simulink model "modellosimulink_sparo"  (R2024b)
settings: Solver=VariableStepAuto  StartTime=0.0  StopTime=10.0  RelTol=1e-3
libraries: arduinolib x29
settings Model: Creator=Andrea Blumer  LastModifiedBy=Andrea Blumer

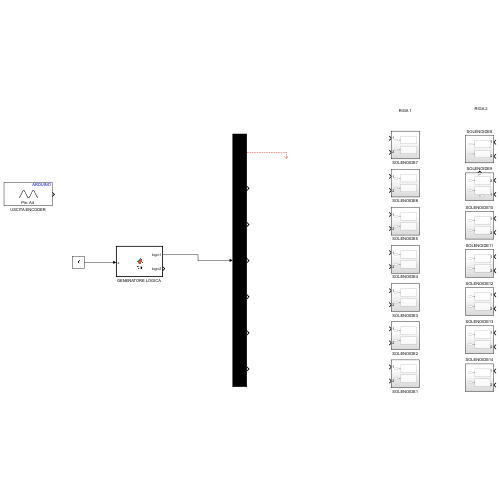
[thumbnail: Simulink's stored preview of the top-level diagram]
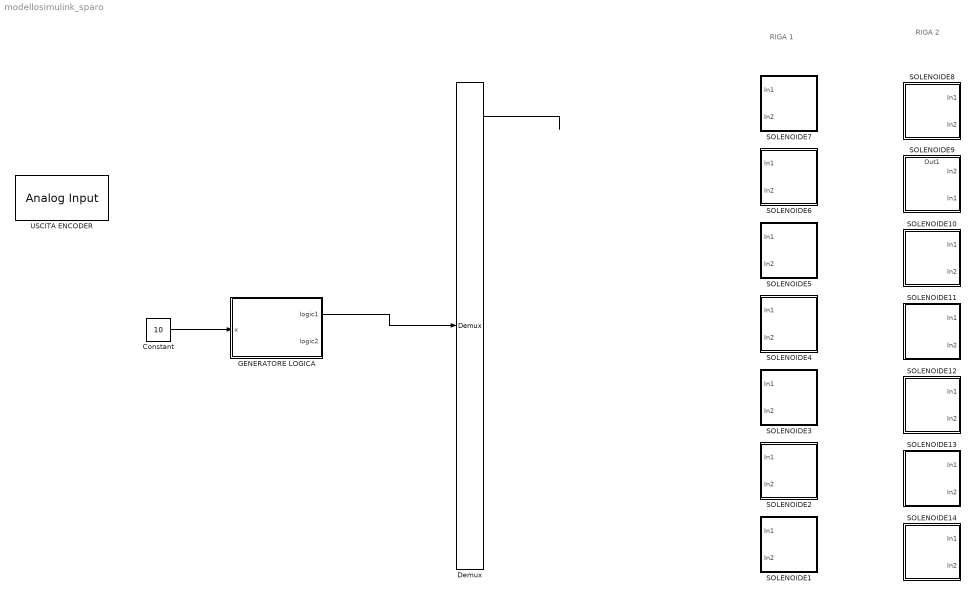
== system modellosimulink_sparo ==
  note: RIGA 1
  note: RIGA 2
  Constant : Constant  Value=10
  Demux : Demux  Outputs=7
  "GENERATORE LOGICA " : MATLAB Function  TreatAsAtomicUnit=on
  SOLENOIDE1 : Subsystem
  SOLENOIDE10 : Subsystem
  SOLENOIDE11 : Subsystem
  SOLENOIDE12 : Subsystem
  SOLENOIDE13 : Subsystem
  SOLENOIDE14 : Subsystem
  SOLENOIDE2 : Subsystem
  SOLENOIDE3 : Subsystem
  SOLENOIDE4 : Subsystem
  SOLENOIDE5 : Subsystem
  SOLENOIDE6 : Subsystem
  SOLENOIDE7 : Subsystem
  SOLENOIDE8 : Subsystem
  SOLENOIDE9 : Subsystem
      settings: PortSchema="{\"entries\":[{\"content\":{\"sides\":[{\"content\":{\"connectorIds\":[\"In1\",\"In2\"]},\"type\":\"ConnectorPlacement.EquallySpacedRectSide\",\"uuid\":\"2699e220-ed49-4c6b-9984-82bf0ed2901a\"},{\"content\":{\"side\":\"RIGHT\"},\"type\":\"ConnectorPlacement.EquallySpacedRectSide\",\"uuid\":\"7975e8f0-8f23-48fb-aa3d-c94205d3d7fe\"},{\"content\":{\"side\":\"TOP\"},\"type\":\"ConnectorPlacement.EquallySpacedRectSide\",\"uuid\":\"15db5694-750a-4b3f-8b7d-6476381e72a2\"},{\"content\":{\"connectorIds\":[\"Out1\"],\"side\":\"BOTTOM\"},\"type\":\"ConnectorPlacement.EquallySpacedRectSide\",\"uuid\":\"d99025a3-6ba6-4f0c-93ef-c9ed91f078e0\"}]},\"type\":\"ConnectorPlacement.EquallySpacedConnector\",\"uuid\":\"e3928348-5078-4e97-9172-3bbb71792ce0\"}],\"packageUris\":[\"http://schema.mathworks.com/mf0/Connector/R2020b\"],\"version\":\"1.0\"}"
  USCITA ENCODER : arduinolib/Analog Input  pinNumber=4  ReadResultsOnly=off  ConversionTriggerSource=Software  ExternalTriggerType=uint32( 0 )  OutputDataType=uint16  EnableConversionCompleteNotify=off  EnableOuputStatus=off  SampleTime=-1  blockPlatform=arduino
      settings: SourceProductName=Common
  wires:
  "GENERATORE LOGICA "/1(logic1) -> Demux/1
  Demux/1 -> ?
  Constant/1 -> "GENERATORE LOGICA "/1(x)

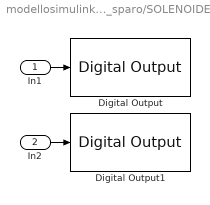
== system modellosimulink_sparo/SOLENOIDE1 ==
  In1 : Inport
  In2 : Inport  Port=2
  Digital Output : arduinolib/Digital Output  pinNumber=9  Direction=output  blockPlatform=arduino
      settings: SourceProductName=Common
  Digital Output1 : arduinolib/Digital Output  pinNumber=9  Direction=output  blockPlatform=arduino
      settings: SourceProductName=Common
  wires:
  In2/1 -> Digital Output1/1
  In1/1 -> Digital Output/1

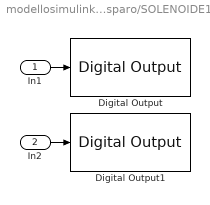
== system modellosimulink_sparo/SOLENOIDE10 ==
  In1 : Inport
  In2 : Inport  Port=2
  Digital Output : arduinolib/Digital Output  pinNumber=9  Direction=output  blockPlatform=arduino
      settings: SourceProductName=Common
  Digital Output1 : arduinolib/Digital Output  pinNumber=9  Direction=output  blockPlatform=arduino
      settings: SourceProductName=Common
  wires:
  In2/1 -> Digital Output1/1
  In1/1 -> Digital Output/1

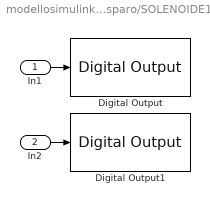
== system modellosimulink_sparo/SOLENOIDE11 ==
  In1 : Inport
  In2 : Inport  Port=2
  Digital Output : arduinolib/Digital Output  pinNumber=9  Direction=output  blockPlatform=arduino
      settings: SourceProductName=Common
  Digital Output1 : arduinolib/Digital Output  pinNumber=9  Direction=output  blockPlatform=arduino
      settings: SourceProductName=Common
  wires:
  In2/1 -> Digital Output1/1
  In1/1 -> Digital Output/1

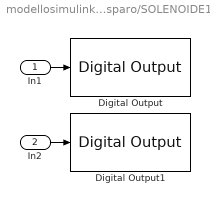
== system modellosimulink_sparo/SOLENOIDE12 ==
  In1 : Inport
  In2 : Inport  Port=2
  Digital Output : arduinolib/Digital Output  pinNumber=9  Direction=output  blockPlatform=arduino
      settings: SourceProductName=Common
  Digital Output1 : arduinolib/Digital Output  pinNumber=9  Direction=output  blockPlatform=arduino
      settings: SourceProductName=Common
  wires:
  In2/1 -> Digital Output1/1
  In1/1 -> Digital Output/1

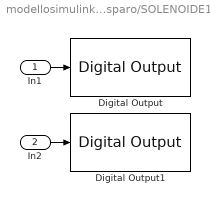
== system modellosimulink_sparo/SOLENOIDE13 ==
  In1 : Inport
  In2 : Inport  Port=2
  Digital Output : arduinolib/Digital Output  pinNumber=9  Direction=output  blockPlatform=arduino
      settings: SourceProductName=Common
  Digital Output1 : arduinolib/Digital Output  pinNumber=9  Direction=output  blockPlatform=arduino
      settings: SourceProductName=Common
  wires:
  In2/1 -> Digital Output1/1
  In1/1 -> Digital Output/1

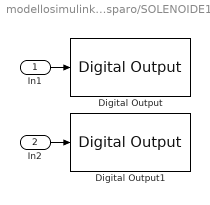
== system modellosimulink_sparo/SOLENOIDE14 ==
  In1 : Inport
  In2 : Inport  Port=2
  Digital Output : arduinolib/Digital Output  pinNumber=9  Direction=output  blockPlatform=arduino
      settings: SourceProductName=Common
  Digital Output1 : arduinolib/Digital Output  pinNumber=9  Direction=output  blockPlatform=arduino
      settings: SourceProductName=Common
  wires:
  In2/1 -> Digital Output1/1
  In1/1 -> Digital Output/1

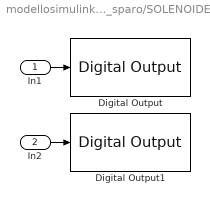
== system modellosimulink_sparo/SOLENOIDE2 ==
  In1 : Inport
  In2 : Inport  Port=2
  Digital Output : arduinolib/Digital Output  pinNumber=9  Direction=output  blockPlatform=arduino
      settings: SourceProductName=Common
  Digital Output1 : arduinolib/Digital Output  pinNumber=9  Direction=output  blockPlatform=arduino
      settings: SourceProductName=Common
  wires:
  In2/1 -> Digital Output1/1
  In1/1 -> Digital Output/1

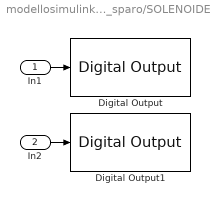
== system modellosimulink_sparo/SOLENOIDE3 ==
  In1 : Inport
  In2 : Inport  Port=2
  Digital Output : arduinolib/Digital Output  pinNumber=9  Direction=output  blockPlatform=arduino
      settings: SourceProductName=Common
  Digital Output1 : arduinolib/Digital Output  pinNumber=9  Direction=output  blockPlatform=arduino
      settings: SourceProductName=Common
  wires:
  In2/1 -> Digital Output1/1
  In1/1 -> Digital Output/1

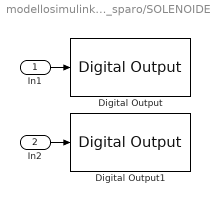
== system modellosimulink_sparo/SOLENOIDE4 ==
  In1 : Inport
  In2 : Inport  Port=2
  Digital Output : arduinolib/Digital Output  pinNumber=9  Direction=output  blockPlatform=arduino
      settings: SourceProductName=Common
  Digital Output1 : arduinolib/Digital Output  pinNumber=9  Direction=output  blockPlatform=arduino
      settings: SourceProductName=Common
  wires:
  In2/1 -> Digital Output1/1
  In1/1 -> Digital Output/1

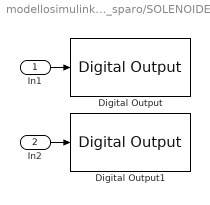
== system modellosimulink_sparo/SOLENOIDE5 ==
  In1 : Inport
  In2 : Inport  Port=2
  Digital Output : arduinolib/Digital Output  pinNumber=9  Direction=output  blockPlatform=arduino
      settings: SourceProductName=Common
  Digital Output1 : arduinolib/Digital Output  pinNumber=9  Direction=output  blockPlatform=arduino
      settings: SourceProductName=Common
  wires:
  In2/1 -> Digital Output1/1
  In1/1 -> Digital Output/1

== system modellosimulink_sparo/SOLENOIDE6 ==
  In1 : Inport
  In2 : Inport  Port=2
  Digital Output : arduinolib/Digital Output  pinNumber=9  Direction=output  blockPlatform=arduino
      settings: SourceProductName=Common
  Digital Output1 : arduinolib/Digital Output  pinNumber=9  Direction=output  blockPlatform=arduino
      settings: SourceProductName=Common
  wires:
  In2/1 -> Digital Output1/1
  In1/1 -> Digital Output/1

== system modellosimulink_sparo/SOLENOIDE7 ==
  In1 : Inport
  In2 : Inport  Port=2
  Digital Output : arduinolib/Digital Output  pinNumber=9  Direction=output  blockPlatform=arduino
      settings: SourceProductName=Common
  Digital Output1 : arduinolib/Digital Output  pinNumber=9  Direction=output  blockPlatform=arduino
      settings: SourceProductName=Common
  wires:
  In2/1 -> Digital Output1/1
  In1/1 -> Digital Output/1

== system modellosimulink_sparo/SOLENOIDE8 ==
  In1 : Inport
  In2 : Inport  Port=2
  Digital Output : arduinolib/Digital Output  pinNumber=9  Direction=output  blockPlatform=arduino
      settings: SourceProductName=Common
  Digital Output1 : arduinolib/Digital Output  pinNumber=9  Direction=output  blockPlatform=arduino
      settings: SourceProductName=Common
  wires:
  In2/1 -> Digital Output1/1
  In1/1 -> Digital Output/1

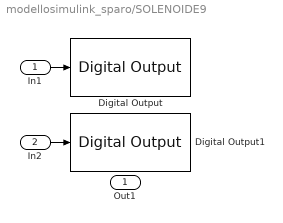
== system modellosimulink_sparo/SOLENOIDE9 ==
  In1 : Inport
  In2 : Inport  Port=2
  Digital Output : arduinolib/Digital Output  pinNumber=9  Direction=output  blockPlatform=arduino
      settings: SourceProductName=Common
  Digital Output1 : arduinolib/Digital Output  pinNumber=9  Direction=output  blockPlatform=arduino
      settings: SourceProductName=Common
  Out1 : Outport
  wires:
  In2/1 -> Digital Output1/1
  In1/1 -> Digital Output/1

== matlab function modellosimulink_sparo/GENERATORE LOGICA  ==
  data: x input; logic1 output; logic2 output
function [logic1, logic2] = fcn(x)
  
    % Carica il file .mat
    data = load('output.mat');

    % Inizializza i vettori di logica per i 7 solenoidi
    logic1 = zeros(1, 7);  % Attrazione
    logic2 = zeros(1, 7);  % Repulsione

    % Trova l'indice della riga che corrisponde al valore di x
    [~, idx] = min(abs(data.X - x));  % Trova l'indice più vicino a x_norm

    % Controlla che l'indice trovato sia valido
    if idx > 0 && idx <= length(data.X)
        % Assegna i valori di attrazione e repulsione per i solenoidi
        coil_attraction = data.COIL_ATTRACTION(idx);  % Valore di attrazione
        coil_repulsion = data.COIL_REPULSION(idx);    % Valore di repulsione
        
        % Imposta i valori nei vettori di logica
        logic1(coil_attraction) = 1;   % Se il solenoide è in attrazione, metti 1
        logic2(coil_repulsion) = -1;    % Se il solenoide è in repulsione, metti -1
    else
        warning('x_norm non trovato nel file output.mat');
    end
end
